simulink subsystem "SAS_PI_slash_D_Controller"  (R2024a)
settings: Solver=VariableStepAuto  StartTime=0.0  StopTime=10.0  RelTol=1e-3
values from neighbouring files (symbols this model uses):
  Kdrr = 0.004    [NCMS_AltMis_Init_항공대.m]
  Kirr = 0.1    [NCMS_AltMis_Init_항공대.m]
  Kprr = 0.1    [NCMS_AltMis_Init_항공대.m]
  Nrr = 50    [NCMS_AltMis_Init_항공대.m]
  SampleTime_SAS = 1/1000    (= 0.001)    [Init_FLIGHT_Hexacopter.m]
libraries: simulink x1, cstblocks x1, slpidlib x1
settings Model: Creator=sslee  LastModifiedBy=sslee

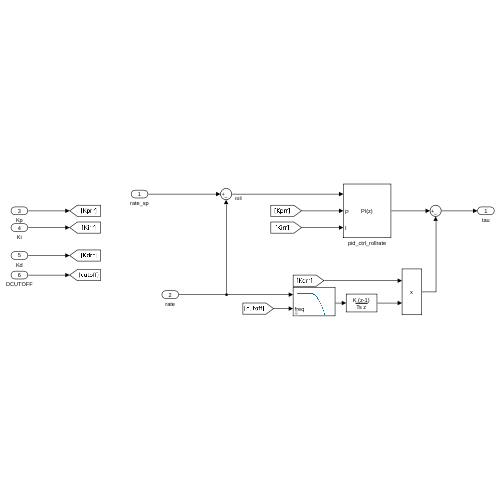
[thumbnail: Simulink's stored preview of the top-level diagram]
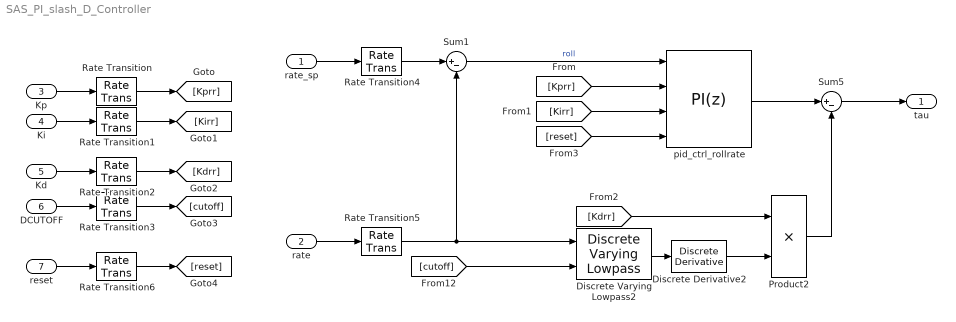
== system SAS_PI_slash_D_Controller ==
  rate_sp : Inport
  rate : Inport  Port=2
  Kp : Inport  Port=3
  Ki : Inport  Port=4
  Kd : Inport  Port=5
  DCUTOFF : Inport  Port=6
  reset : Inport  Port=7
  Discrete Derivative2 : simulink/Discrete/Discrete Derivative  gainval=1.0  ICPrevScaledInput=0.0  OutMin=[]  OutMax=[]  OutDataType=fixdt(1, 16)  OutScaling=2^-10  DoSatur=off
  Discrete Varying Lowpass2 : cstblocks/Linear Parameter Varying/Discrete Varying Lowpass  N=2  w0=0  Ts=SampleTime_SAS
  Product2 : Product
  Rate Transition{,1..6} (7 alike) : RateTransition  OutPortSampleTime=SampleTime_SAS
  Sum1 : Sum  Inputs=|+-
  Sum5 : Sum  Inputs=|+-
  pid_ctrl_rollrate : slpidlib/PID Controller  Controller=PI  Form=Parallel  TimeDomain=Discrete-time  UseExternalTs=off  SampleTime=SampleTime_SAS  IntegratorMethod=Forward Euler  FilterMethod=Forward Euler  ControllerParametersSource=external  P=Kprr  I=Kirr  UseKiTs=off  D=Kdrr  UseExternalDerivativeSource=off  N=Nrr  UseFilter=on  TunerSelectOption=Transfer Function Based (PID Tuner App)  InitialConditionSource=internal  InitialConditionForIntegrator=0  InitialConditionForFilter=0  DifferentiatorICPrevScaledInput=0  ExternalReset=either  TrackingMode=off  Kt=1  LimitOutput=off  SatLimitsSource=internal  UpperSaturationLimit=0.2  LowerSaturationLimit=-0.2  LinearizeAsGain=on  AntiWindupMode=clamping  Kb=1  LimitIntegrator=off  UpperIntegratorSaturationLimit=inf  LowerIntegratorSaturationLimit=-inf  SaturateOnIntegerOverflow=on  POutMin=[]  POutMax=[]  IOutMin=[]  IOutMax=[]  DOutMin=[]  DOutMax=[]  NOutMin=[]  NOutMax=[]  SumOutMin=[]  SumOutMax=[]  SaturationOutDataTypeStr=single  SaturationOutMin=[]  SaturationOutMax=[]  PParamMin=[]  PParamMax=[]  IParamMin=[]  IParamMax=[]  DParamMin=[]  DParamMax=[]  NParamMin=[]  NParamMax=[]  KbParamMin=[]  KbParamMax=[]  KtParamMin=[]  KtParamMax=[]  KbOutMin=[]  KbOutMax=[]  KtOutMin=[]  KtOutMax=[]  IntegratorOutMin=[]  IntegratorOutMax=[]  FilterOutMin=[]  FilterOutMax=[]  SumI1OutMin=[]  SumI1OutMax=[]  SumI2OutMin=[]  SumI2OutMax=[]  SumI3OutMin=[]  SumI3OutMax=[]  SumI4OutMin=[]  SumI4OutMax=[]  SumDOutMin=[]  SumDOutMax=[]  DifferentiatorOutMin=[]  DifferentiatorOutMax=[]  FilterDiffOutCoefMin=[]  FilterDiffOutCoefMax=[]  ReciprocalOutMin=[]  ReciprocalOutMax=[]  SumDenOutMin=[]  SumDenOutMax=[]  SumNumOutMin=[]  SumNumOutMax=[]  DivideOutMin=[]  DivideOutMax=[]  UdiffTsProdOutMin=[]  UdiffTsProdOutMax=[]  NTsProdOutMin=[]  NTsProdOutMax=[]  UintegralTsProdOutMin=[]  UintegralTsProdOutMax=[]  UngainTsProdOutMin=[]  UngainTsProdOutMax=[]  ClampingZeroOutDataTypeStr=Inherit: Inherit via back propagation  ClampingZeroOutMin=[]  ClampingZeroOutMax=[]  FilterDenConstantOutDataTypeStr=Inherit: Inherit via back propagation  FilterDenConstantOutMin=[]  FilterDenConstantOutMax=[]  PCopyOutDataTypeStr=Inherit: Inherit via back propagation  PCopyOutMin=[]  PCopyOutMax=[]  NCopyOutDataTypeStr=Inherit: Inherit via back propagation  NCopyOutMin=[]  NCopyOutMax=[]  IntegratorContinuousStateAttributes=''  IntegratorStateMustResolveToSignalObject=off  IntegratorRTWStateStorageClass=Auto  FilterContinuousStateAttributes=''  FilterStateMustResolveToSignalObject=off  FilterRTWStateStorageClass=Auto  ParallelPVariant=ExternalParameters  IdealPVariant=Disabled  IVariant=ExternalParameters  DVariant=Disabled  IntegratorVariant=Discrete  SatVariant=Disabled  AWVariant=Passthrough  PCopyVariant=Disabled  TRVariant=Disabled  FdbkBlocksVariant=Forward  IdealPFdbkVariant=Disabled  SatFdbkVariant=Disabled  DerivativeFilterVariant=Disabled  NVariant=Disabled  NCopyVariant=Disabled_SignalSpec  FilterICVariant=Disabled  IntegratorICVariant=InternalICs  ExternalResetVariant=ExternalReset  TRSumVariant=Passthrough  SumFdbkVariant=Disabled  SumVariant=Sum_PI  TsampFilterVariant=InternalTs  TsampNgainVariant=Passthrough  TsampIntegralVariant=Disabled_SignalSpec  ExternalSaturationOutDataTypeStr=single  DerivativeSourceVariant=Disabled
  tau : Outport
  wires:
  Sum1/1 -> pid_ctrl_rollrate/1  "roll"
  [Kirr] -> pid_ctrl_rollrate/3
  rate_sp/1 -> Rate Transition4/1
  Product2/1 -> Sum5/2
  Discrete Varying Lowpass2/1 -> Discrete Derivative2/1
  Discrete Derivative2/1 -> Product2/2
  rate/1 -> Rate Transition5/1
  Sum5/1 -> tau/1
  [Kprr] -> pid_ctrl_rollrate/2
  [Kdrr] -> Product2/1
  pid_ctrl_rollrate/1 -> Sum5/1
  Kp/1 -> Rate Transition/1
  Ki/1 -> Rate Transition1/1
  Kd/1 -> Rate Transition2/1
  DCUTOFF/1 -> Rate Transition3/1
  Rate Transition/1 -> [Kprr]
  Rate Transition1/1 -> [Kirr]
  Rate Transition2/1 -> [Kdrr]
  Rate Transition3/1 -> [cutoff]
  Rate Transition4/1 -> Sum1/1
  Rate Transition5/1 -> Sum1/2, Discrete Varying Lowpass2/1
  reset/1 -> Rate Transition6/1
  Rate Transition6/1 -> [reset]
  [reset] -> pid_ctrl_rollrate/4
  [cutoff] -> Discrete Varying Lowpass2/2
